simulink model "threephasexmershortckttest"  (R2024b)
settings: Solver=ode23tb  StartTime=0.0  StopTime=0.1  MaxStep=1e-4  RelTol=1e-3
libraries: spsACVoltageSourceLib x3, spsRMSLib x2, spsGroundLib x1, spsPower3phInstantaneousLib x1, spsThreePhaseTransformerTwoWindingsLib x1, spsThreePhaseVIMeasurementLib x1, sps_lib x1
settings Model: Creator=brain  LastModifiedBy=brain

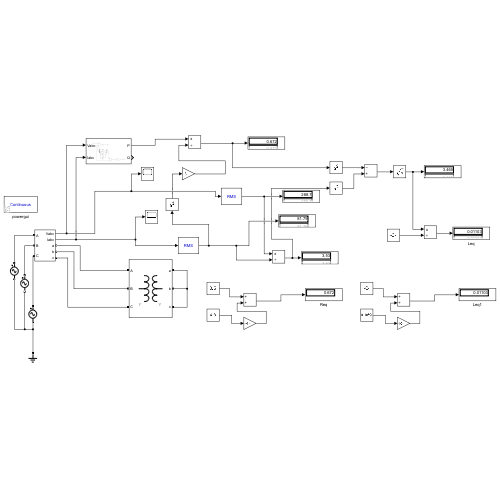
[thumbnail: Simulink's stored preview of the top-level diagram]
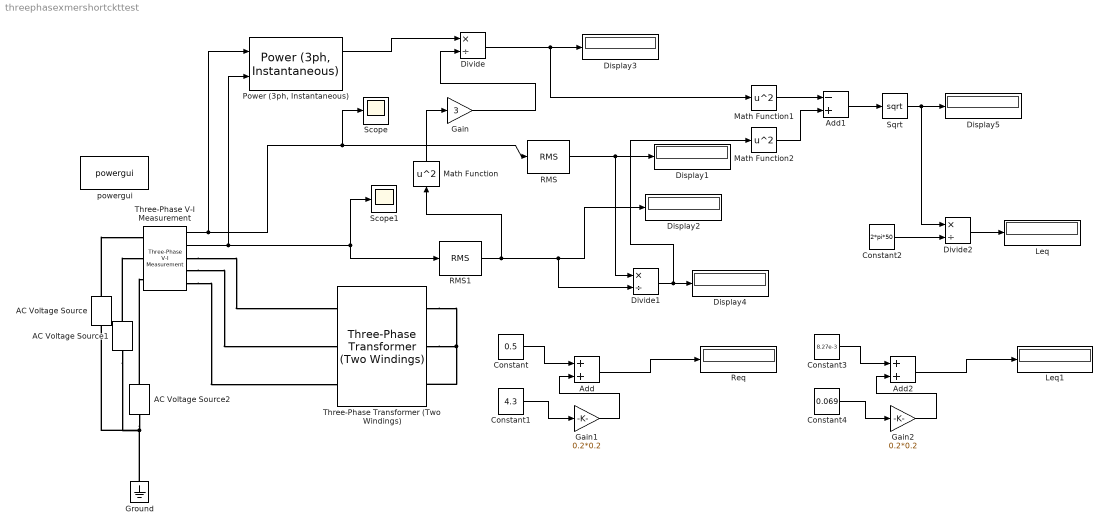
== system threephasexmershortckttest ==
  AC Voltage Source : spsACVoltageSourceLib/AC Voltage Source  Amplitude=0.5*1000*sqrt(2)/sqrt(3)  Phase=0  Frequency=50  SampleTime=0  Measurements=None  BusType=swing  Pref=10e3  Qref=0  Qmin=-inf  Qmax=+inf
  AC Voltage Source1 : spsACVoltageSourceLib/AC Voltage Source  Amplitude=0.5*1000*sqrt(2)/sqrt(3)  Phase=-120  Frequency=50  SampleTime=0  Measurements=None  BusType=swing  Pref=10e3  Qref=0  Qmin=-inf  Qmax=+inf
  AC Voltage Source2 : spsACVoltageSourceLib/AC Voltage Source  Amplitude=0.5*1000*sqrt(2)/sqrt(3)  Phase=120  Frequency=50  SampleTime=0  Measurements=None  BusType=swing  Pref=10e3  Qref=0  Qmin=-inf  Qmax=+inf
  Add : Sum
  Add1 : Sum  Inputs=-+
  Add2 : Sum
  Constant : Constant  Value=0.5
  Constant1 : Constant  Value=4.3
  Constant2 : Constant  Value=2*pi*50
  Constant3 : Constant  Value=8.27e-3
  Constant4 : Constant  Value=0.069
  Display{1..5} (5 alike) : Display
  Divide : Product  Inputs=*/
  Divide1 : Product  Inputs=*/
  Divide2 : Product  Inputs=*/
  Gain : Gain  Gain=3
  Gain1 : Gain  Gain=0.2*0.2
  Gain2 : Gain  Gain=0.2*0.2
  Ground : spsGroundLib/Ground  LConnTagsString=a
  Leq : Display
  Leq1 : Display
  Math Function : Math  Operator=square
  Math Function1 : Math  Operator=square
  Math Function2 : Math  Operator=square
  "Power (3ph, Instantaneous)" : spsPower3phInstantaneousLib/Power (3ph, Instantaneous)
  RMS : spsRMSLib/RMS  TrueRMS=off  Freq=50  RMSInit=0  Ts=0
  RMS1 : spsRMSLib/RMS  TrueRMS=off  Freq=50  RMSInit=0  Ts=0
  Req : Display
  Scope : Scope
  Scope1 : Scope
  Sqrt : Sqrt
  Three-Phase Transformer (Two Windings) : spsThreePhaseTransformerTwoWindingsLib/Three-Phase Transformer (Two Windings)  Winding1Connection=Y  Winding2Connection=Y  CoreType=Three single-phase transformers  SetSaturation=off  Hysteresis=off  DataFile='hysteresis'  SetInitialFlux=off  Measurements=None  UNITS=SI  NominalPower=[ 2000e3 , 50 ]  Winding1=[6.6e3 0.5 8.27e-3]  Winding2=[33e3 4.3 0.069]  Rm=10000  Lm=500  L0=0.034664  Saturation=[0 0;0.59382 20.584;247.42 26.073]  InitialFluxes=[13.723 -13.723 12.007]  BreakLoop=off  DiscreteSolver=Trapezoidal iterative  DataType=on  TransfoNumber=1
  Three-Phase V-I Measurement : spsThreePhaseVIMeasurementLib/Three-Phase V-I Measurement  VoltageMeasurement=phase-to-ground  SetLabelV=off  LabelV=Vabc  Vpu=off  VpuLL=off  CurrentMeasurement=yes  SetLabelI=off  LabelI=Iabc  Ipu=off  Pbase=100e6  Vbase=500e3  OutputType=Complex  PhasorSimulation=off  PSBequivalent=0
  powergui : sps_lib/powergui  Priority=1  SimulationMode=Continuous  SampleTime=50e-6  frequency=60  Iterations=50  frequencyindice=50  Pbase=100e6  ErrMax=1e-4  UnitsV=kV  UnitsW=MW  buscounter=0  FunctionMessages=off  echomessages=off  EnableUseOfTLC=off  CurrentSourceSwitches=off  DisableSnubberDevices=off  DisableRonSwitches=off  DisableVfSwitches=off  DisplayEquations=off  AutomaticDiscreteSolvers=off  SolverType=Tustin/Backward Euler (TBE)  Interpol=off  ExternalGateDelay=off  methode=off  Ts=100  x0status=blocks  SPID=on  SwTol=0  HookPort=off  NonlinearTolerance=1e-4  nMaxIteration=100  ContinueOnMaxIteration=off  RestoreLinks=warning  ResistiveCurrentMeasurement=off  Frange=[0:2:500]  Ylog=off  Xlog=on  ShowGrid=off  save=off  variable=ZData  structure=0  ZoomFFT=off  StartTime=0.0  cycles=1  DisplayStyle=1  fundamental=60  FreqAxis=off  MaxFrequency=1000  frequencyindicesteady=1  RmsSteady=1  display=off
  wires:
  Three-Phase V-I Measurement/1 -> "Power (3ph, Instantaneous)"/1, Scope/1, RMS/1
  Three-Phase V-I Measurement/2 -> "Power (3ph, Instantaneous)"/2, RMS1/1, Scope1/1
  RMS1/1 -> Divide1/2, Display2/1, Math Function/1
  RMS/1 -> Divide1/1, Display1/1
  Gain/1 -> Divide/2
  Math Function/1 -> Gain/1
  Constant/1 -> Add/1
  Constant1/1 -> Gain1/1
  Gain1/1 -> Add/2
  Add/1 -> Req/1
  "Power (3ph, Instantaneous)"/1 -> Divide/1
  Divide1/1 -> Math Function2/1, Display4/1
  Divide/1 -> Math Function1/1, Display3/1
  Math Function1/1 -> Add1/1
  Math Function2/1 -> Add1/2
  Add1/1 -> Sqrt/1
  Sqrt/1 -> Divide2/1, Display5/1
  Constant2/1 -> Divide2/2
  Divide2/1 -> Leq/1
  Add2/1 -> Leq1/1
  Gain2/1 -> Add2/2
  Constant4/1 -> Gain2/1
  Constant3/1 -> Add2/1
  connections:
  AC Voltage Source2/LConn1 -- AC Voltage Source1/LConn1 -- AC Voltage Source/LConn1 -- Ground/LConn1
  AC Voltage Source/RConn1 -- Three-Phase V-I Measurement/LConn1
  AC Voltage Source1/RConn1 -- Three-Phase V-I Measurement/LConn2
  AC Voltage Source2/RConn1 -- Three-Phase V-I Measurement/LConn3
  Three-Phase V-I Measurement/RConn1 -- Three-Phase Transformer (Two Windings)/LConn1
  Three-Phase V-I Measurement/RConn2 -- Three-Phase Transformer (Two Windings)/LConn2
  Three-Phase V-I Measurement/RConn3 -- Three-Phase Transformer (Two Windings)/LConn3
  Three-Phase Transformer (Two Windings)/RConn1 -- Three-Phase Transformer (Two Windings)/RConn2 -- Three-Phase Transformer (Two Windings)/RConn3
